simulink library "IGSI_lib"  (Simulink 7.5)
settings: Solver=ode45  StartTime=0.0  StopTime=10.0  RelTol=1e-3
values from neighbouring files (symbols this model uses):
  pSHLI_bool_ImmoCheckEnbl = Simulink.Parameter    [IGSI_par.m]
undefined symbols (not defined in the file or in its folder): ImmoModTyp, p_bool_True_M
libraries: BaseOperationLib_Browser x6, PES_CZ_FAW x2, simulink x1
settings Model: Creator=wuaibin  LastModifiedBy=wuaibin

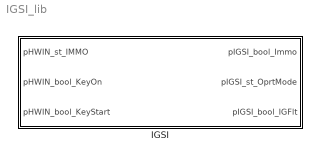
== system IGSI_lib ==
  IGSI : Subsystem  TreatAsAtomicUnit=on

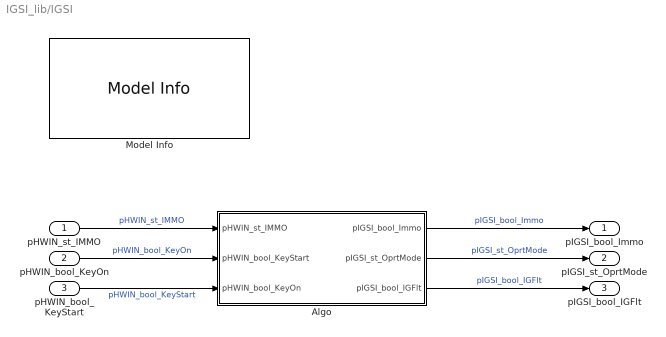
== system IGSI_lib/IGSI ==
  pHWIN_st_IMMO : Inport  OutDataType=fixdt(1, 16)  OutScaling=2^0
  pHWIN_bool_KeyOn : Inport  Port=2  OutDataType=fixdt(1, 16)  OutScaling=2^0
  pHWIN_bool_KeyStart : Inport  Port=3  OutDataType=fixdt(1, 16)  OutScaling=2^0
  Algo : Subsystem
  Model Info : simulink/Model-Wide Utilities/Model Info  SystemSampleTime=-1  InitialBlockCM=None  BlockCM=None  Frame=on  DisplayStringWithTags=Model Info\nCreated: %<Created>\nCreator: zhangqiang  HorizontalTextAlignment=Center  LeftAlignmentValue=0.5  SourceBlockDiagram=HQEV_HCU  TagMaxNumber=20
  pIGSI_bool_Immo : Outport  OutDataType=fixdt(1, 16)  OutScaling=2^0
  pIGSI_st_OprtMode : Outport  Port=2  OutDataType=fixdt(1, 16)  OutScaling=2^0
  pIGSI_bool_IGFlt : Outport  Port=3  OutDataType=fixdt(1, 16)  OutScaling=2^0
  wires:
  pHWIN_st_IMMO/1 -> Algo/1(pHWIN_st_IMMO)  "pHWIN_st_IMMO"
  Algo/2(pIGSI_st_OprtMode) -> pIGSI_st_OprtMode/1  "pIGSI_st_OprtMode"
  pHWIN_bool_KeyOn/1 -> Algo/2(pHWIN_bool_KeyStart)  "pHWIN_bool_KeyOn"
  pHWIN_bool_KeyStart/1 -> Algo/3(pHWIN_bool_KeyOn)  "pHWIN_bool_KeyStart"
  Algo/3(pIGSI_bool_IGFlt) -> pIGSI_bool_IGFlt/1  "pIGSI_bool_IGFlt"
  Algo/1(pIGSI_bool_Immo) -> pIGSI_bool_Immo/1  "pIGSI_bool_Immo"

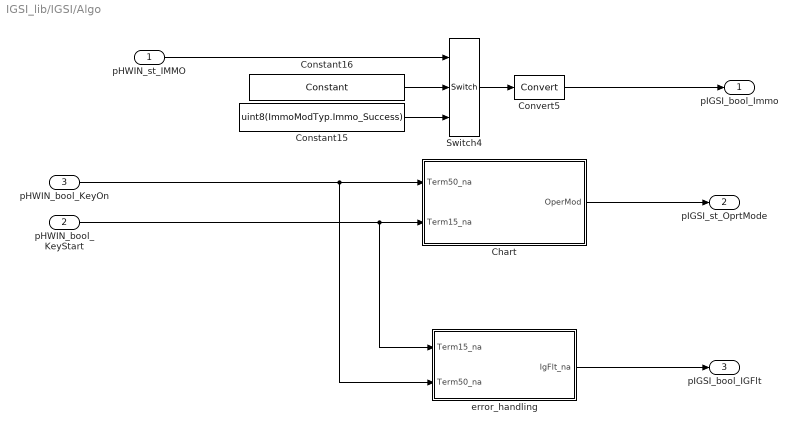
== system IGSI_lib/IGSI/Algo ==
  pHWIN_st_IMMO : Inport  OutDataType=fixdt(1, 16)  OutScaling=2^0
  pHWIN_bool_KeyStart : Inport  Port=2  OutDataType=fixdt(1, 16)  OutScaling=2^0
  pHWIN_bool_KeyOn : Inport  Port=3  OutDataType=fixdt(1, 16)  OutScaling=2^0
  Chart : Stateflow chart  TreatAsAtomicUnit=on
  Constant15 : Constant  Value=uint8(ImmoModTyp.Immo_Success)  OutDataTypeMode=uint8  OutDataType=fixdt(1, 16)  OutScaling=2^0  OutDataTypeStr=uint8
  Constant16 : BaseOperationLib_Browser/Sources&Sinks/Constant  Value=pSHLI_bool_ImmoCheckEnbl  OutMin=[]  OutMax=[]  OutDataType=fixdt(1, 16)  ConRadixGroup=Use specified scaling  OutScaling=2^0  OutDataTypeStr=Inherit: Inherit from 'Constant value'
  Convert5 : DataTypeConversion  OutDataType=fixdt(1, 16)  OutScaling=2^0
  Switch4 : BaseOperationLib_Browser/Signal Routing Changed/Switch  Criteria=u2 ~= 0  Threshold=1  InputSameDT=on  OutMin=[]  OutMax=[]  OutDataType=fixdt(1,16,0)  OutScaling=[]  SaturateOnIntegerOverflow=on
  error_handling : Subsystem
  pIGSI_bool_Immo : Outport  OutDataType=fixdt(1, 16)  OutScaling=2^0
  pIGSI_st_OprtMode : Outport  Port=2  OutDataType=fixdt(1, 16)  OutScaling=2^0
  pIGSI_bool_IGFlt : Outport  Port=3  OutDataType=fixdt(1, 16)  OutScaling=2^0
  wires:
  Switch4/1 -> Convert5/1
  pHWIN_st_IMMO/1 -> Switch4/1
  Constant16/1 -> Switch4/2
  Constant15/1 -> Switch4/3
  Convert5/1 -> pIGSI_bool_Immo/1
  pHWIN_bool_KeyStart/1 -> error_handling/1(Term15_na), Chart/2(Term15_na)
  pHWIN_bool_KeyOn/1 -> error_handling/2(Term50_na), Chart/1(Term50_na)
  Chart/1(OperMod) -> pIGSI_st_OprtMode/1
  error_handling/1(IgFlt_na) -> pIGSI_bool_IGFlt/1

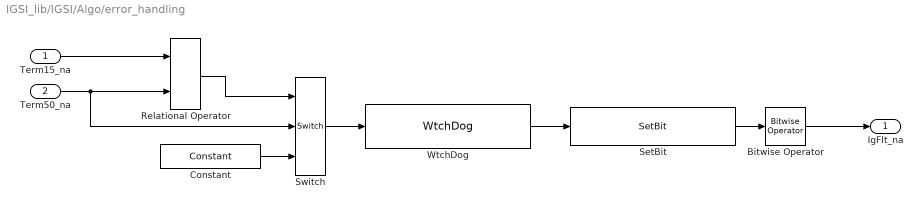
== system IGSI_lib/IGSI/Algo/error_handling ==
  Term15_na : Inport
  Term50_na : Inport  Port=2
  Bitwise Operator : BaseOperationLib_Browser/Others Unchanged/Bitwise Operator  logicop=OR  UseBitMask=off  BitMask=bin2dec('11011001')  BitMaskRealWorld=Stored Integer
  Constant : BaseOperationLib_Browser/Sources&Sinks/Constant  Value=p_bool_True_M  OutMin=[]  OutMax=[]  OutDataType=fixdt(1, 16)  ConRadixGroup=Use specified scaling  OutScaling=2^0  OutDataTypeStr=Inherit: Inherit from 'Constant value'
  Relational Operator : BaseOperationLib_Browser/Logic Operations Changed/Relational Operator  Operator===  InputSameDT=on  LogicOutDataTypeMode=Specify via dialog  LogicDataType=PDT_Bool  OutDataTypeStr=PDT_Bool
  SetBit : PES_CZ_FAW/Discontinuities/SetBit  SystemSampleTime=-1  maska=FltTypIGSI.T50T15TiOut_ERR
  Switch : BaseOperationLib_Browser/Signal Routing Changed/Switch  Criteria=u2 ~= 0  Threshold=1  InputSameDT=on  OutMin=[]  OutMax=[]  OutDataType=fixdt(1,16,0)  OutScaling=[]  SaturateOnIntegerOverflow=on
  WtchDog : PES_CZ_FAW/Discontinuities/WtchDog  SystemSampleTime=-1  timeoutthres=p_IGSI_Term50Term15Tiout_s
  IgFlt_na : Outport
  wires:
  Relational Operator/1 -> Switch/1
  Constant/1 -> Switch/3
  Switch/1 -> WtchDog/1
  WtchDog/1 -> SetBit/1
  SetBit/1 -> Bitwise Operator/1
  Term15_na/1 -> Relational Operator/1
  Term50_na/1 -> Switch/2, Relational Operator/2
  Bitwise Operator/1 -> IgFlt_na/1

== stateflow chart IGSI/Algo/Chart ==
  state Terminal_15
    en:
    OperMod = OperModTyp.CL15;
  state Ignition_off
    en:
    OperMod = OperModTyp.IG_OFF;
  state Terminal_50
    en:
    OperMod = OperModTyp.CL50;
  (default) -> Ignition_off
  Ignition_off -> Terminal_15 : [Term15_na]
  Terminal_15 -> Terminal_50 [order 2] : [Term50_na]
  Terminal_50 -> Ignition_off [order 1] : [!Term15_na]
  Terminal_15 -> Ignition_off [order 1] : [!Term15_na && ...
      | !Term50_na]
  Terminal_50 -> Terminal_15 [order 2] : [!Term50_na]
  data: Term50_na input double; Term15_na input double; OperMod output uint8
